simulink model "ReachTask_SensoryConfound"  (R2022b)
settings: Solver=FixedStepDiscrete  StartTime=0.0  StopTime=10  FixedStep=0.001  RelTol=1e-3  EnableMultiTasking=on
PreLoadFcn:
  | parambus = Simulink.Bus;
  | idx = 0;
  | 
  | idx = idx + 1;
  | parambus.Elements(idx) = Simulink.BusElement;
  | parambus.Elements(idx).Name = 'ScreenOn';
  | parambus.Elements(idx).DataType = 'uint8';
  | parambus.Elements(idx).Dimensions = [1, 1];
  | 
  | idx = idx + 1;
  | parambus.Elements(idx) = Simulink.BusElement;
  | parambus.Elements(idx).Name = 'DelayPeriod';
  | parambus.Elements(idx).DataType = 'uint16';
  | parambus.Elements(idx).Dimensions = [1, 2];
  | 
  | idx = idx + 1;
  | parambus.Elements(idx) = Simulink.BusElement;
  | parambus.Elements(idx).Name = 'TargetHoldTime';
  | parambus.Elements(idx).DataType = 'uint16';
  | parambus.Elements(idx).Dimensions = [1, 1];
  | 
  | idx = idx + 1;
  | parambus.Elements(idx) = Simulink.BusElement;
  | parambus.Elements(idx).Name = 'TrialTimeout';
  | parambus.Elements(idx).DataType = 'uint16';
  | parambus.Elements(idx).Dimensions = [1, 1];
settings Model: Creator=irwin  LastModifiedBy=irwin
settings SolverCC: ConcurrentTasks=on  AlgebraicLoopSolver=TrustRegion  PositivePriorityOrder=on  InsertRTBMode=Never (minimum delay)
settings DataIOCC: SaveFormat=Array  SaveState=on  SignalLoggingName=logsOut
settings OptimizationCC: BlockReduction=off  BooleanDataType=off  OptimizeBlockIOStorage=off  BufferReuse=off  GlobalBufferReuse=off  ExpressionFolding=off  LocalBlockOutputs=off  InitFltsAndDblsToZero=on  OptimizeDataStoreBuffers=off  BusAssignmentInplaceUpdate=off
settings DebuggingCC: SaveWithParameterizedLinksMsg=none  UnderspecifiedInitializationDetection=Classic  MergeDetectMultiDrivingBlocksExec=none  CheckExecutionContextPreStartOutputMsg=on  SignalResolutionControl=TryResolveAllWithWarning  TasksWithSamePriorityMsg=none  UnconnectedInputMsg=warning  UnconnectedOutputMsg=warning  UnconnectedLineMsg=warning  SFUnexpectedBacktrackingDiag=warning  SFNoUnconditionalDefaultTransitionDiag=warning  SFExecutionAtInitializationDiag=none  SFMachineParentedDataDiag=warning  ArithmeticOperatorsInVariantConditions=warning
settings HardwareCC: ProdBitPerLong=64  ProdLongLongMode=on  ProdHWDeviceType=Intel->x86-64 (Linux 64)
settings ModelReferenceCC: EnableRefExpFcnMdlSchedulingChecks=on  PropagateSignalLabelsOutOfModel=off
settings SFSimCC: SimUseLocalCustomCode=off  SimTargetLang=C++
settings RTWCC: Description=Simulink Real-Time  SystemTargetFile=slrealtime.tlc  TemplateMakefile=slrealtime_default_tmf  RTWUseLocalCustomCode=off  Toolchain=Simulink Real-Time Toolchain  BuildConfiguration=Faster Runs  CodeExecutionProfiling=on  TargetLang=C++  DLArmComputeVersion=19.05
settings CodeAppCC: StateflowObjectComments=on
settings SimulinkRealTimeTargetCC: MATLABClassNameForMDSCustomization=Simulink.SoftwareTarget.GRTCustomization  UseGCCFastMath=on
settings ConfigComp: CovMetricSettings=dw  CovSaveCumulativeToWorkspaceVar=on  CovSaveSingleToWorkspaceVar=on  CovExternalEMLEnable=off  CovSFcnEnable=off

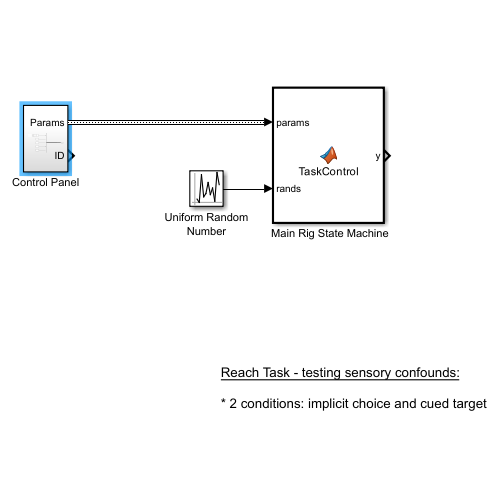
[thumbnail: Simulink's stored preview of the top-level diagram]
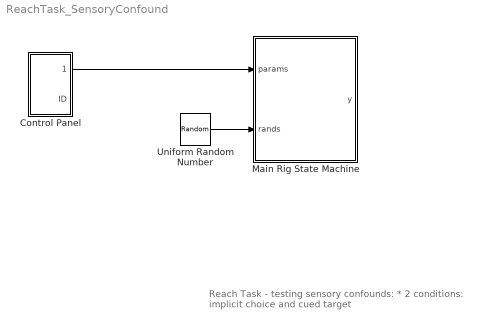
== system ReachTask_SensoryConfound ==
  note: Reach Task - testing sensory confounds:
      |
      | * 2 conditions: implicit choice and cued target
  " Main Rig State Machine" : MATLAB Function  TreatAsAtomicUnit=on
  Control Panel : Subsystem
  Uniform Random Number : UniformRandomNumber  Minimum=[0, 0, 0]  Maximum=[2, 2, 1]  SampleTime=0.1
  wires:
  Uniform Random Number/1 -> " Main Rig State Machine"/2(rands)
  Control Panel/1(Params) -> " Main Rig State Machine"/1(params)

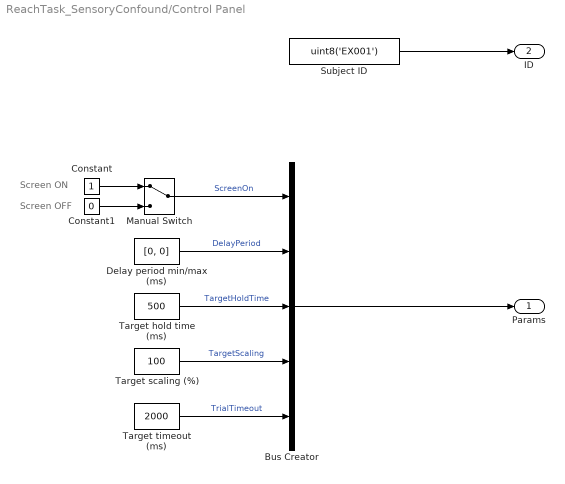
== system ReachTask_SensoryConfound/Control Panel ==
  note: Screen ON
  note: Screen OFF
  Bus Creator : BusCreator  Inputs=5  OutDataTypeStr=Bus: parambus  NonVirtualBus=on
      settings: InheritFromInputs=off
  Constant : Constant  OutDataTypeStr=uint8
  Constant1 : Constant  Value=0  OutDataTypeStr=uint8
  Delay period min/max (ms) : Constant  Value=[0, 0]  OutDataTypeStr=uint16
  Manual Switch : ManualSwitch
  Subject ID : Constant  Value=uint8('EX001')  OutDataTypeStr=uint8
  Target hold time (ms) : Constant  Value=500  OutDataTypeStr=uint16
  Target scaling (%) : Constant  Value=100  OutDataTypeStr=uint8
  Target timeout (ms) : Constant  Value=2000  OutDataTypeStr=uint16
  Params : Outport
  ID : Outport  Port=2
  wires:
  Delay period min/max (ms)/1 -> Bus Creator/2  "DelayPeriod"
  Manual Switch/1 -> Bus Creator/1  "ScreenOn"
  Constant1/1 -> Manual Switch/2
  Constant/1 -> Manual Switch/1
  Bus Creator/1 -> Params/1
  Target hold time (ms)/1 -> Bus Creator/3  "TargetHoldTime"
  Subject ID/1 -> ID/1
  Target timeout (ms)/1 -> Bus Creator/5  "TrialTimeout"
  Target scaling (%)/1 -> Bus Creator/4  "TargetScaling"

== matlab function ReachTask_SensoryConfound/ Main Rig State Machine ==
  data: params input; rands input; y output
function y = TaskControl(params, rands)

persistent exp_state trial_state exp_time trial_time trial_count intparams extparams

if (isempty(exp_state))
    exp_state = uint8(0);           % Experiment state variable
    trial_state = uint8(0);         % Trial state variable
    exp_time = uint32(-1);          % Current experiment time
    trial_time = uint32(0);         % Current trial time
    trial_count = uint16(0);        % Count of the trials in the current run
    extparams = params;             % Initialize parameters to incoming struct

    intparams = struct('TrialType', uint8(0), ...   % 2 trial conditions - implicit/cued
                       'Target', uint8(0), ...      % 2 targets - left/right
                       'DelayTime', uint16(0));     % delay period (ms)

end

%%%%%%%%%%%%%%%%%%%%%%%%%%%%%%% Defines %%%%%%%%%%%%%%%%%%%%%%%%%%%%%%%%%%%

% Trial states:
tstate = struct('INIT',  uint8(0), ...
                'HOME',  uint8(1), ...
                'DELAY', uint8(2), ...
                'REACH', uint8(3), ...
                'HOLD',  uint8(4), ...
                'DONE',  uint8(5));

%%%%%%%%%%%%%%%%%%%%%%%%% Per-timestep updates %%%%%%%%%%%%%%%%%%%%%%%%%%%%

exp_time = exp_time + 1;     % Update simulation time (1 ms per function call)
trial_time = trial_time + 1; % Update trial time

%%%%%%%%%%%%%%%%%%%%%%% Stateflow switch statement %%%%%%%%%%%%%%%%%%%%%%%%

switch exp_state % Primary taskflow (experiment)
    case 0      % Initializing the File Logger
        
        exp_state = uint8(1);
    case 1      % Run the experiment
        switch trial_state % Secondary taskflow (per trial)

            case tstate.INIT

                %Pick up changes to trial parameters:
                extparams = params;
                
                % Determine whether this trial will be cued or not:
                intparams.TrialType = uint8(floor(rands(1))); % 0 = implicit choice, 1 = cued
                
                % If cued, determine target:
                if (intparams.TrialType == 0)
                    intparams.Target = uint8(255);
                else
                    intparams.Target = uint8(floor(rands(2)));
                end
                
                % Determine delay period time:
                intparams.DelayTime = round(rands(3)*diff(extparams.DelayPeriod) + extparams.DelayPeriod(1));

                trial_state = tstate.HOME;
                trial_count = trial_count + uint16(1);
                trial_time = uint32(0);

            case tstate.HOME

                %%% Test for cursor in home target and complete hold
                
                trial_state = tstate.DELAY;

            case tstate.DELAY

            case tstate.DONE
                trial_state = uint8(0);

        end
end


%%%%%%%%%%%%%%%%%%%%%%%% Assign Output Variables: %%%%%%%%%%%%%%%%%%%%%%%%%

y = 1;


end
